simulink model "system_MW"  (R2023b)
settings: Solver=VariableStepAuto  StartTime=0.0  StopTime=0.3  MaxStep=1e-3  RelTol=1e-3  AbsTol=1e-3  EnableMultiTasking=on
values from neighbouring files (symbols this model uses):
  Ts = ts(k)    [example_MW.m]
  Un = 400    [example_MW.m]
undefined symbols (not defined in the file or in its folder): P
libraries: fl_lib x41, nesl_utility x27, ee_lib x19, eeGeneralControl x8
(part 1 of 2)
settings Model: Creator=neugebch  LastModifiedBy=neugebch
settings SolverCC: AutoScaleAbsTol=off  AlgebraicLoopSolver=TrustRegion  MaxZcPerStep=1
settings DataIOCC: LimitDataPoints=on  MaxDataPoints=10000
settings OptimizationCC: ReuseModelBlockBuffer=off  LifeSpan=inf
settings DebuggingCC: UnconnectedInputMsg=warning  UnconnectedOutputMsg=warning  UnconnectedLineMsg=warning  AllowSymbolicDim=off  SFUnexpectedBacktrackingDiag=warning  SFNoUnconditionalDefaultTransitionDiag=warning  SFExecutionAtInitializationDiag=none  ArithmeticOperatorsInVariantConditions=warning
settings ModelReferenceCC: EnableRefExpFcnMdlSchedulingChecks=on
settings SFSimCC: SimUseLocalCustomCode=off  CustomCodeUndefinedFunction=UseInterfaceOnly
settings RTWCC: RTWUseLocalCustomCode=off  DLArmComputeVersion=19.05
settings CodeAppCC: StateflowObjectComments=on
settings GRTTargetCC: TargetLangStandard=C89/C90 (ANSI)
settings ConfigComp: CovMetricSettings=dw  CovSaveCumulativeToWorkspaceVar=on  CovSaveSingleToWorkspaceVar=on  CovExternalEMLEnable=off  CovSFcnEnable=off
settings SimscapeCC: SimscapeLogType=all  SimscapeLogSimulationStatistics=on  SimscapeLogDataHistory=10000

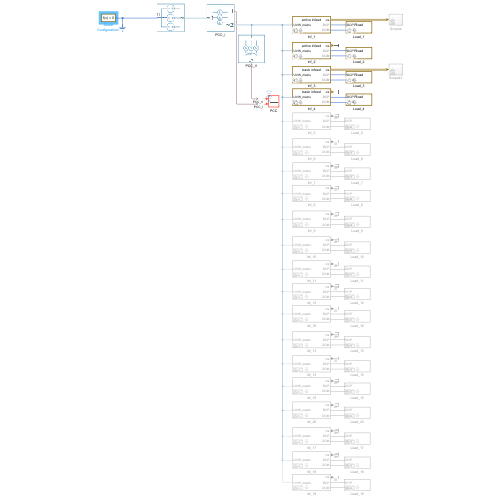
[thumbnail: Simulink's stored preview of the top-level diagram]
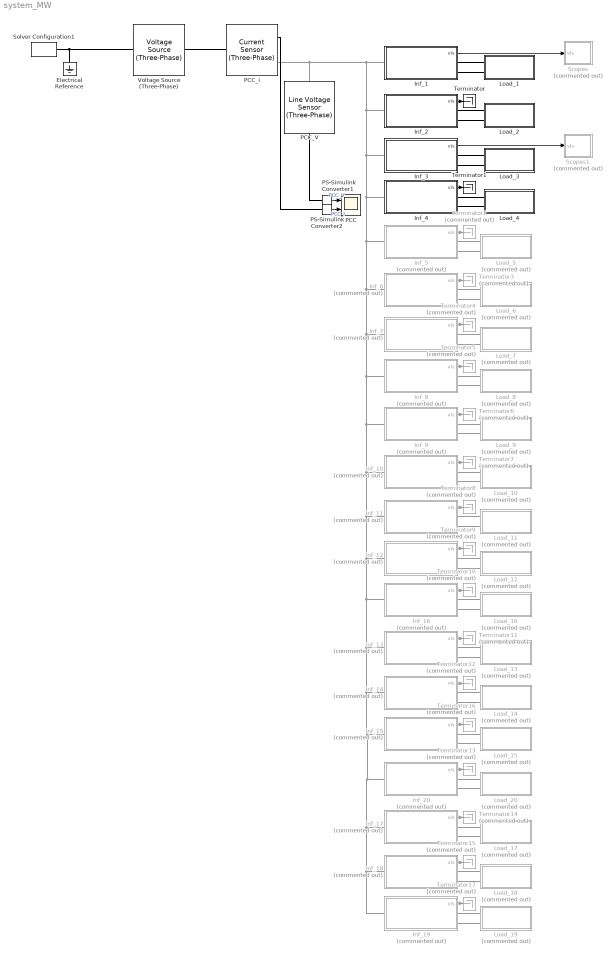
== system system_MW ==
  Electrical Reference : fl_lib/Electrical/Electrical Elements/Electrical Reference
  Inf_1 : Subsystem  Variant=on  mask{P=P(1), Ts=Ts}
  Inf_10 : Subsystem  Commented=on  Variant=on  mask{P=P(10), Ts=Ts}
  Inf_11 : Subsystem  Commented=on  Variant=on  mask{P=P(11), Ts=Ts}
  Inf_12 : Subsystem  Commented=on  Variant=on  mask{P=P(12), Ts=Ts}
  Inf_13 : Subsystem  Commented=on  Variant=on  mask{P=P(14), Ts=Ts}
  Inf_14 : Subsystem  Commented=on  Variant=on  mask{P=P(15), Ts=Ts}
  Inf_15 : Subsystem  Commented=on  Variant=on  mask{P=P(16), Ts=Ts}
  Inf_16 : Subsystem  Commented=on  Variant=on  mask{P=P(13), Ts=Ts}
  Inf_17 : Subsystem  Commented=on  Variant=on  mask{P=P(18), Ts=Ts}
  Inf_18 : Subsystem  Commented=on  Variant=on  mask{P=P(19), Ts=Ts}
  Inf_19 : Subsystem  Commented=on  Variant=on  mask{P=P(20), Ts=Ts}
  Inf_2 : Subsystem  Variant=on  mask{P=P(2), Ts=Ts}
  Inf_20 : Subsystem  Commented=on  Variant=on  mask{P=P(17), Ts=Ts}
  Inf_3 : Subsystem  Variant=on  mask{P=P(3), Ts=Ts}
  Inf_4 : Subsystem  Variant=on  mask{P=P(4), Ts=Ts}
  Inf_5 : Subsystem  Commented=on  Variant=on  mask{P=P(5), Ts=Ts}
  Inf_6 : Subsystem  Commented=on  Variant=on  mask{P=P(6), Ts=Ts}
  Inf_7 : Subsystem  Commented=on  Variant=on  mask{P=P(7), Ts=Ts}
  Inf_8 : Subsystem  Commented=on  Variant=on  mask{P=P(8), Ts=Ts}
  Inf_9 : Subsystem  Commented=on  Variant=on  mask{P=P(9), Ts=Ts}
  Load_1 : Subsystem  Variant=on  mask{P=P(1)}
  Load_10 : Subsystem  Commented=on  Variant=on  mask{P=P(10)}
  Load_11 : Subsystem  Commented=on  Variant=on  mask{P=P(11)}
  Load_12 : Subsystem  Commented=on  Variant=on  mask{P=P(12)}
  Load_13 : Subsystem  Commented=on  Variant=on  mask{P=P(14)}
  Load_14 : Subsystem  Commented=on  Variant=on  mask{P=P(15)}
  Load_15 : Subsystem  Commented=on  Variant=on  mask{P=P(16)}
  Load_16 : Subsystem  Commented=on  Variant=on  mask{P=P(13)}
  Load_17 : Subsystem  Commented=on  Variant=on  mask{P=P(18)}
  Load_18 : Subsystem  Commented=on  Variant=on  mask{P=P(19)}
  Load_19 : Subsystem  Commented=on  Variant=on  mask{P=P(20)}
  Load_2 : Subsystem  Variant=on  mask{P=P(2)}
  Load_20 : Subsystem  Commented=on  Variant=on  mask{P=P(17)}
  Load_3 : Subsystem  Variant=on  mask{P=P(3)}
  Load_4 : Subsystem  Variant=on  mask{P=P(4)}
  Load_5 : Subsystem  Commented=on  Variant=on  mask{P=P(5)}
  Load_6 : Subsystem  Commented=on  Variant=on  mask{P=P(6)}
  Load_7 : Subsystem  Commented=on  Variant=on  mask{P=P(7)}
  Load_8 : Subsystem  Commented=on  Variant=on  mask{P=P(8)}
  Load_9 : Subsystem  Commented=on  Variant=on  mask{P=P(9)}
  PCC : Scope  NumInputPorts=2
  PCC_V : ee_lib/Sensors & Transducers/Line Voltage Sensor (Three-Phase)
      settings: LogSimulationData=on
  PCC_i : ee_lib/Sensors & Transducers/Current Sensor (Three-Phase)
      settings: LogSimulationData=on
  PS-Simulink Converter1 : nesl_utility/PS-Simulink Converter  PhysicalDomain=network_engine_domain  SubClassName=ps_output  LeftPortType=input  RightPortType=output  PseudoPeriodic=off  Frequencies=[]  VectorFormat=inherit  Unit=inherit  AffineConversion=off
  PS-Simulink Converter2 : nesl_utility/PS-Simulink Converter  PhysicalDomain=network_engine_domain  SubClassName=ps_output  LeftPortType=input  RightPortType=output  PseudoPeriodic=off  Frequencies=[]  VectorFormat=inherit  Unit=inherit  AffineConversion=off
  Scopes : Subsystem  Commented=on
  Scopes1 : Subsystem  Commented=on
  Solver Configuration1 : nesl_utility/Solver Configuration  PhysicalDomain=network_engine_domain  SubClassName=solver  LeftPortType=input  RightPortType=generic  Tones=[]  Harmonics=[]  SimulateNoise=off  Profile=off  UseLocalSampling=off  EnableSwitchedLinearOptims=on  FrequencyDomain=off  UseCCode=off  RelTol=0.001  AbsTol=1e-06  MinStep=1e-09  ToWorkspace=off  RevertToSquareIcSolve=off  NumHomotopyIterations=100  PhasorMode=off  PhasorModeNumHarmonics=1  ConsistencySolver=NEWTON_FTOL  IndexReductionMethod=DerivativeReplacement  DoDC=off  ResidualTolerance=1e-09  ConsistencyTolSource=GLOBAL  ConsistencyAbsTol=0.001  ConsistencyRelTol=0.001  ConsistencyTolFactor=0.001  UseLocalSolver=on  LocalSolverChoice=NE_TRAPEZOIDAL_ADVANCER  ResolveIndetEquations=on  FunctionEvalNumThread=1  LocalSolverSampleTime=Ts  DoFixedCost=on  MaxNonlinIter=5  MaxModeIter=2  ComputeImpulses=off  ImpulseIterations=1  LinearAlgebra=auto  LinearAlgebraNumThread=0  EquationFormulation=NE_TIME_EF  DelaysMemoryBudget=1024  AutomaticFiltering=on  FilteringTimeConstant=0.001  PartitionStorageMethod=AS_NEEDED  PartitionMemoryBudget=1024  PartitionMethod=ROBUST  MultibodyUseLocalSolver=off  MultibodyLocalSolverChoice=ODE1  MultibodyLocalSolverSampleTime=0.001
  Terminator : Terminator
  Terminator1 : Terminator
  Terminator{2..17} (16 alike) : Terminator  Commented=on
  Voltage Source (Three-Phase) : ee_lib/Sources/Voltage Source (Three-Phase)  vline_rms=sqrt(3/2) * Un V  shift=0 deg  freq=fn Hz  impedance_option=1  SShortCircuit=Skv A*V  XR=X_R  R=0.01 Ohm  L=3.97e-4 H  harmonic_option=0  harmonic_orders=[5, 7, 11, 13]  harmonic_ratios=[.1, .1, .1, .1]  G_parasitic=0 1/Ohm  I_specify=off  I_priority=None  I=[0, 0, 0] A  I_nominal_specify=off  I_nominal_unit=A  I_nominal_value=1
  wires:
  Inf_1/1(vis) -> Scopes/1(vis)
  Inf_3/1(vis) -> Scopes1/1(vis)
  PS-Simulink Converter1/1 -> PCC/1  "PCC_V"
  PS-Simulink Converter2/1 -> PCC/2  "PCC_I"
  Inf_2/1(vis) -> Terminator/1
  Inf_4/1(vis) -> Terminator1/1
  Inf_5/1(vis) -> Terminator2/1
  Inf_6/1(vis) -> Terminator3/1
  Inf_7/1(vis) -> Terminator4/1
  Inf_8/1(vis) -> Terminator5/1
  Inf_9/1(vis) -> Terminator6/1
  Inf_10/1(vis) -> Terminator7/1
  Inf_11/1(vis) -> Terminator8/1
  Inf_12/1(vis) -> Terminator9/1
  Inf_16/1(vis) -> Terminator10/1
  Inf_13/1(vis) -> Terminator11/1
  Inf_14/1(vis) -> Terminator12/1
  Inf_15/1(vis) -> Terminator16/1
  Inf_20/1(vis) -> Terminator13/1
  Inf_17/1(vis) -> Terminator14/1
  Inf_18/1(vis) -> Terminator15/1
  Inf_19/1(vis) -> Terminator17/1
  connections:
  Solver Configuration1/RConn1 -- Voltage Source (Three-Phase)/LConn1 -- Electrical Reference/LConn1
  Inf_18/LConn1 -- Inf_20/LConn1 -- Inf_14/LConn1 -- Inf_13/LConn1 -- Inf_10/LConn1 -- Inf_7/LConn1 -- Inf_2/LConn1 -- PCC_V/LConn1 -- PCC_i/RConn2 -- Inf_1/LConn1 -- Inf_3/LConn1 -- Inf_4/LConn1 -- Inf_5/LConn1 -- Inf_6/LConn1 -- Inf_8/LConn1 -- Inf_9/LConn1 -- Inf_11/LConn1 -- Inf_12/LConn1 -- Inf_16/LConn1 -- Inf_15/LConn1 -- Inf_17/LConn1 -- Inf_19/LConn1
  PS-Simulink Converter1/LConn1 -- PCC_V/RConn1
  Load_1/LConn1 -- Inf_1/RConn1
  Load_1/LConn2 -- Inf_1/RConn2
  Load_2/LConn1 -- Inf_2/RConn1
  Load_2/LConn2 -- Inf_2/RConn2
  Load_3/LConn1 -- Inf_3/RConn1
  Load_3/LConn2 -- Inf_3/RConn2
  Voltage Source (Three-Phase)/RConn1 -- PCC_i/LConn1
  PS-Simulink Converter2/LConn1 -- PCC_i/RConn1
  Load_4/LConn2 -- Inf_4/RConn2
  Load_4/LConn1 -- Inf_4/RConn1
  Load_8/LConn1 -- Inf_8/RConn1
  Load_6/LConn2 -- Inf_6/RConn2
  Inf_5/RConn2 -- Load_5/LConn2
  Load_6/LConn1 -- Inf_6/RConn1
  Load_7/LConn2 -- Inf_7/RConn2
  Load_8/LConn2 -- Inf_8/RConn2
  Inf_5/RConn1 -- Load_5/LConn1
  Load_7/LConn1 -- Inf_7/RConn1
  Load_11/LConn1 -- Inf_11/RConn1
  Inf_9/RConn1 -- Load_9/LConn1
  Load_10/LConn1 -- Inf_10/RConn1
  Load_12/LConn2 -- Inf_12/RConn2
  Load_11/LConn2 -- Inf_11/RConn2
  Inf_9/RConn2 -- Load_9/LConn2
  Load_12/LConn1 -- Inf_12/RConn1
  Load_10/LConn2 -- Inf_10/RConn2
  Load_13/LConn2 -- Inf_13/RConn2
  Load_15/LConn1 -- Inf_15/RConn1
  Load_14/LConn2 -- Inf_14/RConn2
  Inf_16/RConn2 -- Load_16/LConn2
  Load_15/LConn2 -- Inf_15/RConn2
  Load_13/LConn1 -- Inf_13/RConn1
  Load_14/LConn1 -- Inf_14/RConn1
  Inf_16/RConn1 -- Load_16/LConn1
  Inf_20/RConn1 -- Load_20/LConn1
  Load_19/LConn2 -- Inf_19/RConn2
  Inf_20/RConn2 -- Load_20/LConn2
  Load_17/LConn1 -- Inf_17/RConn1
  Load_18/LConn2 -- Inf_18/RConn2
  Load_17/LConn2 -- Inf_17/RConn2
  Load_19/LConn1 -- Inf_19/RConn1
  Load_18/LConn1 -- Inf_18/RConn1

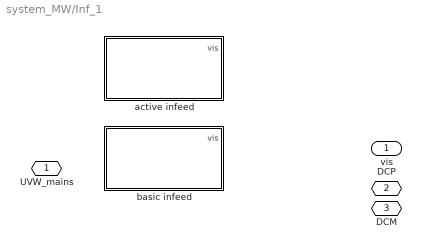
== system system_MW/Inf_1 ==
  active infeed : Subsystem  Variant=on  VariantControlMode=label  VariantControl=true  LabelModeActiveChoice=Choice
  basic infeed : Subsystem  Variant=on  VariantControlMode=label  VariantControl=false  LabelModeActiveChoice=Choice_1
  UVW_mains : PMIOPort  Side=Left
  DCP : PMIOPort  Port=2  Side=Right
  DCM : PMIOPort  Port=3  Side=Right
  vis : Outport

== system system_MW/Inf_10 ==
  active infeed : Subsystem  VariantControl=true  ReferencedSubsystem=active_infeed  P=P  Ts=Ts
  basic infeed : Subsystem  VariantControl=false  ReferencedSubsystem=basic_infeed  P=P  Ts=Ts
  UVW_mains : PMIOPort  Side=Left
  DCP : PMIOPort  Port=2  Side=Right
  DCM : PMIOPort  Port=3  Side=Right
  vis : Outport

== system system_MW/Inf_11 ==
  active infeed : Subsystem  VariantControl=false  ReferencedSubsystem=active_infeed  P=P  Ts=Ts
  basic infeed : Subsystem  VariantControl=true  ReferencedSubsystem=basic_infeed  P=P  Ts=Ts
  UVW_mains : PMIOPort  Side=Left
  DCP : PMIOPort  Port=2  Side=Right
  DCM : PMIOPort  Port=3  Side=Right
  vis : Outport

== system system_MW/Inf_12 ==
  active infeed : Subsystem  VariantControl=false  ReferencedSubsystem=active_infeed  P=P  Ts=Ts
  basic infeed : Subsystem  VariantControl=true  ReferencedSubsystem=basic_infeed  P=P  Ts=Ts
  UVW_mains : PMIOPort  Side=Left
  DCP : PMIOPort  Port=2  Side=Right
  DCM : PMIOPort  Port=3  Side=Right
  vis : Outport

== system system_MW/Inf_13 ==
  active infeed : Subsystem  VariantControl=true  ReferencedSubsystem=active_infeed  P=P  Ts=Ts
  basic infeed : Subsystem  VariantControl=false  ReferencedSubsystem=basic_infeed  P=P  Ts=Ts
  UVW_mains : PMIOPort  Side=Left
  DCP : PMIOPort  Port=2  Side=Right
  DCM : PMIOPort  Port=3  Side=Right
  vis : Outport

== system system_MW/Inf_14 ==
  active infeed : Subsystem  VariantControl=false  ReferencedSubsystem=active_infeed  P=P  Ts=Ts
  basic infeed : Subsystem  VariantControl=true  ReferencedSubsystem=basic_infeed  P=P  Ts=Ts
  UVW_mains : PMIOPort  Side=Left
  DCP : PMIOPort  Port=2  Side=Right
  DCM : PMIOPort  Port=3  Side=Right
  vis : Outport

== system system_MW/Inf_15 ==
  active infeed : Subsystem  VariantControl=false  ReferencedSubsystem=active_infeed  P=P  Ts=Ts
  basic infeed : Subsystem  VariantControl=true  ReferencedSubsystem=basic_infeed  P=P  Ts=Ts
  UVW_mains : PMIOPort  Side=Left
  DCP : PMIOPort  Port=2  Side=Right
  DCM : PMIOPort  Port=3  Side=Right
  vis : Outport

== system system_MW/Inf_16 ==
  active infeed : Subsystem  Variant=on  VariantControlMode=label  VariantControl=true  LabelModeActiveChoice=Choice
  basic infeed : Subsystem  Variant=on  VariantControlMode=label  VariantControl=false  LabelModeActiveChoice=Choice_1
  UVW_mains : PMIOPort  Side=Left
  DCP : PMIOPort  Port=2  Side=Right
  DCM : PMIOPort  Port=3  Side=Right
  vis : Outport

== system system_MW/Inf_17 ==
  active infeed : Subsystem  VariantControl=true  ReferencedSubsystem=active_infeed  P=P  Ts=Ts
  basic infeed : Subsystem  VariantControl=false  ReferencedSubsystem=basic_infeed  P=P  Ts=Ts
  UVW_mains : PMIOPort  Side=Left
  DCP : PMIOPort  Port=2  Side=Right
  DCM : PMIOPort  Port=3  Side=Right
  vis : Outport

== system system_MW/Inf_18 ==
  active infeed : Subsystem  VariantControl=false  ReferencedSubsystem=active_infeed  P=P  Ts=Ts
  basic infeed : Subsystem  VariantControl=true  ReferencedSubsystem=basic_infeed  P=P  Ts=Ts
  UVW_mains : PMIOPort  Side=Left
  DCP : PMIOPort  Port=2  Side=Right
  DCM : PMIOPort  Port=3  Side=Right
  vis : Outport

== system system_MW/Inf_19 ==
  active infeed : Subsystem  VariantControl=false  ReferencedSubsystem=active_infeed  P=P  Ts=Ts
  basic infeed : Subsystem  VariantControl=true  ReferencedSubsystem=basic_infeed  P=P  Ts=Ts
  UVW_mains : PMIOPort  Side=Left
  DCP : PMIOPort  Port=2  Side=Right
  DCM : PMIOPort  Port=3  Side=Right
  vis : Outport

== system system_MW/Inf_2 ==
  active infeed : Subsystem  VariantControl=true  ReferencedSubsystem=active_infeed  P=P  Ts=Ts
  basic infeed : Subsystem  VariantControl=false  ReferencedSubsystem=basic_infeed  P=P  Ts=Ts
  UVW_mains : PMIOPort  Side=Left
  DCP : PMIOPort  Port=2  Side=Right
  DCM : PMIOPort  Port=3  Side=Right
  vis : Outport

== system system_MW/Inf_20 ==
  active infeed : Subsystem  Variant=on  VariantControlMode=label  VariantControl=true  LabelModeActiveChoice=Choice
  basic infeed : Subsystem  Variant=on  VariantControlMode=label  VariantControl=false  LabelModeActiveChoice=Choice_1
  UVW_mains : PMIOPort  Side=Left
  DCP : PMIOPort  Port=2  Side=Right
  DCM : PMIOPort  Port=3  Side=Right
  vis : Outport

== system system_MW/Inf_3 ==
  active infeed : Subsystem  VariantControl=false  ReferencedSubsystem=active_infeed  P=P  Ts=Ts
  basic infeed : Subsystem  VariantControl=true  ReferencedSubsystem=basic_infeed  P=P  Ts=Ts
  UVW_mains : PMIOPort  Side=Left
  DCP : PMIOPort  Port=2  Side=Right
  DCM : PMIOPort  Port=3  Side=Right
  vis : Outport

== system system_MW/Inf_4 ==
  active infeed : Subsystem  VariantControl=false  ReferencedSubsystem=active_infeed  P=P  Ts=Ts
  basic infeed : Subsystem  VariantControl=true  ReferencedSubsystem=basic_infeed  P=P  Ts=Ts
  UVW_mains : PMIOPort  Side=Left
  DCP : PMIOPort  Port=2  Side=Right
  DCM : PMIOPort  Port=3  Side=Right
  vis : Outport

== system system_MW/Inf_5 ==
  active infeed : Subsystem  Variant=on  VariantControlMode=label  VariantControl=true  LabelModeActiveChoice=Choice
  basic infeed : Subsystem  Variant=on  VariantControlMode=label  VariantControl=false  LabelModeActiveChoice=Choice_1
  UVW_mains : PMIOPort  Side=Left
  DCP : PMIOPort  Port=2  Side=Right
  DCM : PMIOPort  Port=3  Side=Right
  vis : Outport

== system system_MW/Inf_6 ==
  active infeed : Subsystem  VariantControl=true  ReferencedSubsystem=active_infeed  P=P  Ts=Ts
  basic infeed : Subsystem  VariantControl=false  ReferencedSubsystem=basic_infeed  P=P  Ts=Ts
  UVW_mains : PMIOPort  Side=Left
  DCP : PMIOPort  Port=2  Side=Right
  DCM : PMIOPort  Port=3  Side=Right
  vis : Outport

== system system_MW/Inf_7 ==
  active infeed : Subsystem  VariantControl=false  ReferencedSubsystem=active_infeed  P=P  Ts=Ts
  basic infeed : Subsystem  VariantControl=true  ReferencedSubsystem=basic_infeed  P=P  Ts=Ts
  UVW_mains : PMIOPort  Side=Left
  DCP : PMIOPort  Port=2  Side=Right
  DCM : PMIOPort  Port=3  Side=Right
  vis : Outport

== system system_MW/Inf_8 ==
  active infeed : Subsystem  VariantControl=false  ReferencedSubsystem=active_infeed  P=P  Ts=Ts
  basic infeed : Subsystem  VariantControl=true  ReferencedSubsystem=basic_infeed  P=P  Ts=Ts
  UVW_mains : PMIOPort  Side=Left
  DCP : PMIOPort  Port=2  Side=Right
  DCM : PMIOPort  Port=3  Side=Right
  vis : Outport

== system system_MW/Inf_9 ==
  active infeed : Subsystem  Variant=on  VariantControlMode=label  VariantControl=true  LabelModeActiveChoice=Choice
  basic infeed : Subsystem  Variant=on  VariantControlMode=label  VariantControl=false  LabelModeActiveChoice=Choice_1
  UVW_mains : PMIOPort  Side=Left
  DCP : PMIOPort  Port=2  Side=Right
  DCM : PMIOPort  Port=3  Side=Right
  vis : Outport

== system system_MW/Load_1 ==
  Rload : Subsystem  VariantControl=true  ReferencedSubsystem=Rload
  Vdc : Subsystem  VariantControl=false  ReferencedSubsystem=Vdc
  DCP : PMIOPort  Side=Left
  DCM : PMIOPort  Port=2  Side=Left

== system system_MW/Load_10 ==
  Rload : Subsystem  VariantControl=true
  Vdc : Subsystem  VariantControl=false
  DCP : PMIOPort  Side=Left
  DCM : PMIOPort  Port=2  Side=Left

== system system_MW/Load_11 ==
  Rload : Subsystem  VariantControl=true
  Vdc : Subsystem  VariantControl=false
  DCP : PMIOPort  Side=Left
  DCM : PMIOPort  Port=2  Side=Left

== system system_MW/Load_12 ==
  Rload : Subsystem  VariantControl=true
  Vdc : Subsystem  VariantControl=false
  DCP : PMIOPort  Side=Left
  DCM : PMIOPort  Port=2  Side=Left

== system system_MW/Load_13 ==
  Rload : Subsystem  VariantControl=true
  Vdc : Subsystem  VariantControl=false
  DCP : PMIOPort  Side=Left
  DCM : PMIOPort  Port=2  Side=Left

== system system_MW/Load_14 ==
  Rload : Subsystem  VariantControl=true
  Vdc : Subsystem  VariantControl=false
  DCP : PMIOPort  Side=Left
  DCM : PMIOPort  Port=2  Side=Left

== system system_MW/Load_15 ==
  Rload : Subsystem  VariantControl=true
  Vdc : Subsystem  VariantControl=false
  DCP : PMIOPort  Side=Left
  DCM : PMIOPort  Port=2  Side=Left

== system system_MW/Load_16 ==
  Rload : Subsystem  VariantControl=true
  Vdc : Subsystem  VariantControl=false
  DCP : PMIOPort  Side=Left
  DCM : PMIOPort  Port=2  Side=Left

== system system_MW/Load_17 ==
  Rload : Subsystem  VariantControl=true
  Vdc : Subsystem  VariantControl=false
  DCP : PMIOPort  Side=Left
  DCM : PMIOPort  Port=2  Side=Left

== system system_MW/Load_18 ==
  Rload : Subsystem  VariantControl=true
  Vdc : Subsystem  VariantControl=false
  DCP : PMIOPort  Side=Left
  DCM : PMIOPort  Port=2  Side=Left

== system system_MW/Load_19 ==
  Rload : Subsystem  VariantControl=true
  Vdc : Subsystem  VariantControl=false
  DCP : PMIOPort  Side=Left
  DCM : PMIOPort  Port=2  Side=Left

== system system_MW/Load_2 ==
  Rload : Subsystem  VariantControl=true  ReferencedSubsystem=Rload
  Vdc : Subsystem  VariantControl=false  ReferencedSubsystem=Vdc
  DCP : PMIOPort  Side=Left
  DCM : PMIOPort  Port=2  Side=Left

== system system_MW/Load_20 ==
  Rload : Subsystem  VariantControl=true
  Vdc : Subsystem  VariantControl=false
  DCP : PMIOPort  Side=Left
  DCM : PMIOPort  Port=2  Side=Left

== system system_MW/Load_3 ==
  Rload : Subsystem  VariantControl=true  ReferencedSubsystem=Rload
  Vdc : Subsystem  VariantControl=false  ReferencedSubsystem=Vdc
  DCP : PMIOPort  Side=Left
  DCM : PMIOPort  Port=2  Side=Left

== system system_MW/Load_4 ==
  Rload : Subsystem  VariantControl=true  ReferencedSubsystem=Rload
  Vdc : Subsystem  VariantControl=false  ReferencedSubsystem=Vdc
  DCP : PMIOPort  Side=Left
  DCM : PMIOPort  Port=2  Side=Left

== system system_MW/Load_5 ==
  Rload : Subsystem  VariantControl=true
  Vdc : Subsystem  VariantControl=false
  DCP : PMIOPort  Side=Left
  DCM : PMIOPort  Port=2  Side=Left

== system system_MW/Load_6 ==
  Rload : Subsystem  VariantControl=true
  Vdc : Subsystem  VariantControl=false
  DCP : PMIOPort  Side=Left
  DCM : PMIOPort  Port=2  Side=Left

== system system_MW/Load_7 ==
  Rload : Subsystem  VariantControl=true
  Vdc : Subsystem  VariantControl=false
  DCP : PMIOPort  Side=Left
  DCM : PMIOPort  Port=2  Side=Left

== system system_MW/Load_8 ==
  Rload : Subsystem  VariantControl=true
  Vdc : Subsystem  VariantControl=false
  DCP : PMIOPort  Side=Left
  DCM : PMIOPort  Port=2  Side=Left

== system system_MW/Load_9 ==
  Rload : Subsystem  VariantControl=true
  Vdc : Subsystem  VariantControl=false
  DCP : PMIOPort  Side=Left
  DCM : PMIOPort  Port=2  Side=Left

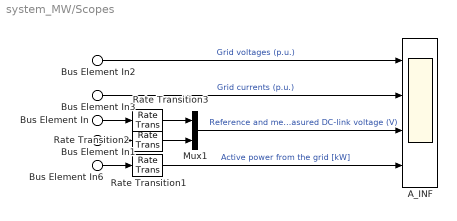
== system system_MW/Scopes ==
  Bus Element In : Inport  PortName=vis  Element=VdcRef
  Bus Element In1 : Inport  PortName=vis  Element=VdcF
  Bus Element In2 : Inport  PortName=vis  Element=VgABC
  Bus Element In3 : Inport  PortName=vis  Element=IgABC
  Bus Element In6 : Inport  PortName=vis  Element=Pt
  A_INF : Scope  NumInputPorts=4
  Mux1 : Mux  Inputs=2
  Rate Transition1 : RateTransition
  Rate Transition2 : RateTransition
  Rate Transition3 : RateTransition
  wires:
  Rate Transition2/1 -> Mux1/2
  Bus Element In/1 -> Rate Transition3/1
  Mux1/1 -> A_INF/3  "Reference and measured DC-link voltage (V)"
  Bus Element In2/1 -> A_INF/1  "Grid voltages (p.u.)"
  Bus Element In3/1 -> A_INF/2  "Grid currents (p.u.)"
  Rate Transition1/1 -> A_INF/4  "Active power from the grid [kW]"
  Bus Element In1/1 -> Rate Transition2/1
  Rate Transition3/1 -> Mux1/1
  Bus Element In6/1 -> Rate Transition1/1

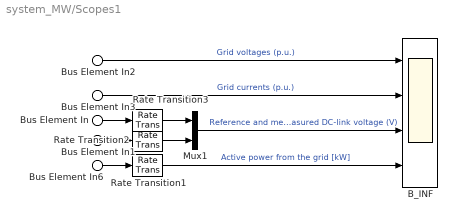
== system system_MW/Scopes1 ==
  Bus Element In : Inport  PortName=vis  Element=VdcRef
  Bus Element In1 : Inport  PortName=vis  Element=VdcF
  Bus Element In2 : Inport  PortName=vis  Element=VgABC
  Bus Element In3 : Inport  PortName=vis  Element=IgABC
  Bus Element In6 : Inport  PortName=vis  Element=Pt
  B_INF : Scope  NumInputPorts=4
  Mux1 : Mux  Inputs=2
  Rate Transition1 : RateTransition
  Rate Transition2 : RateTransition
  Rate Transition3 : RateTransition
  wires:
  Bus Element In6/1 -> Rate Transition1/1
  Rate Transition3/1 -> Mux1/1
  Bus Element In1/1 -> Rate Transition2/1
  Rate Transition1/1 -> B_INF/4  "Active power from the grid [kW]"
  Bus Element In3/1 -> B_INF/2  "Grid currents (p.u.)"
  Bus Element In2/1 -> B_INF/1  "Grid voltages (p.u.)"
  Mux1/1 -> B_INF/3  "Reference and measured DC-link voltage (V)"
  Bus Element In/1 -> Rate Transition3/1
  Rate Transition2/1 -> Mux1/2

== system system_MW/Inf_1/active infeed ==
  active infeed : Subsystem  VariantControl=Choice  ReferencedSubsystem=active_infeed  P=P  Ts=Ts
  UVW_mains : PMIOPort  Side=Left
  DCP : PMIOPort  Port=2  Side=Right
  DCM : PMIOPort  Port=3  Side=Right
  vis : Outport

== system system_MW/Inf_1/basic infeed ==
  basic infeed : Subsystem  VariantControl=Choice_1  ReferencedSubsystem=basic_infeed  P=P  Ts=Ts
  UVW_mains : PMIOPort  Side=Left
  DCP : PMIOPort  Port=2  Side=Right
  DCM : PMIOPort  Port=3  Side=Right
  vis : Outport

== system system_MW/Inf_16/active infeed ==
  active infeed : Subsystem  VariantControl=Choice  ReferencedSubsystem=active_infeed  P=P  Ts=Ts
  UVW_mains : PMIOPort  Side=Left
  DCP : PMIOPort  Port=2  Side=Right
  DCM : PMIOPort  Port=3  Side=Right
  vis : Outport

== system system_MW/Inf_16/basic infeed ==
  basic infeed : Subsystem  VariantControl=Choice_1  ReferencedSubsystem=basic_infeed  P=P  Ts=Ts
  UVW_mains : PMIOPort  Side=Left
  DCP : PMIOPort  Port=2  Side=Right
  DCM : PMIOPort  Port=3  Side=Right
  vis : Outport

== system system_MW/Inf_20/active infeed ==
  active infeed : Subsystem  VariantControl=Choice  ReferencedSubsystem=active_infeed  P=P  Ts=Ts
  UVW_mains : PMIOPort  Side=Left
  DCP : PMIOPort  Port=2  Side=Right
  DCM : PMIOPort  Port=3  Side=Right
  vis : Outport

== system system_MW/Inf_20/basic infeed ==
  basic infeed : Subsystem  VariantControl=Choice_1  ReferencedSubsystem=basic_infeed  P=P  Ts=Ts
  UVW_mains : PMIOPort  Side=Left
  DCP : PMIOPort  Port=2  Side=Right
  DCM : PMIOPort  Port=3  Side=Right
  vis : Outport

== system system_MW/Inf_5/active infeed ==
  active infeed : Subsystem  VariantControl=Choice  ReferencedSubsystem=active_infeed  P=P  Ts=Ts
  UVW_mains : PMIOPort  Side=Left
  DCP : PMIOPort  Port=2  Side=Right
  DCM : PMIOPort  Port=3  Side=Right
  vis : Outport

== system system_MW/Inf_5/basic infeed ==
  basic infeed : Subsystem  VariantControl=Choice_1  ReferencedSubsystem=basic_infeed  P=P  Ts=Ts
  UVW_mains : PMIOPort  Side=Left
  DCP : PMIOPort  Port=2  Side=Right
  DCM : PMIOPort  Port=3  Side=Right
  vis : Outport

== system system_MW/Inf_9/active infeed ==
  active infeed : Subsystem  VariantControl=Choice  ReferencedSubsystem=active_infeed  P=P  Ts=Ts
  UVW_mains : PMIOPort  Side=Left
  DCP : PMIOPort  Port=2  Side=Right
  DCM : PMIOPort  Port=3  Side=Right
  vis : Outport

== system system_MW/Inf_9/basic infeed ==
  basic infeed : Subsystem  VariantControl=Choice_1  ReferencedSubsystem=basic_infeed  P=P  Ts=Ts
  UVW_mains : PMIOPort  Side=Left
  DCP : PMIOPort  Port=2  Side=Right
  DCM : PMIOPort  Port=3  Side=Right
  vis : Outport

== system system_MW/Load_10/Rload ==
  Resistor1 : fl_lib/Electrical/Electrical Elements/Resistor  R=P.Un/P.In/P.p Ohm  i_specify=off  i_priority=None  i=0 A  i_nominal_specify=off  i_nominal_unit=A  i_nominal_value=1  v_specify=off  v_priority=None  v=0 V  v_nominal_specify=off  v_nominal_unit=V  v_nominal_value=1
  DCP : PMIOPort  Side=Left
  DCM : PMIOPort  Port=2  Side=Left
  connections:
  DCM/RConn1 -- Resistor1/RConn1
  DCP/RConn1 -- Resistor1/LConn1

== system system_MW/Load_10/Vdc ==
  Voltage Source : ee_lib/Sources/Voltage Source  dc_voltage=P.Udc V  ac_voltage=0 V  ac_shift=0 rad  ac_frequency=fn Hz  noise_mode=ee.enum.sources.noise.Disabled  PSD=0 V^2/Hz  sample_time=1e-3 s  repeatability=ee.enum.sources.repeatability.NotRepeatable  user_seed=0  auto_seed=3346497771  i_specify=off  i_priority=None  i=0 A  i_nominal_specify=off  i_nominal_unit=A  i_nominal_value=1  v_specify=off  v_priority=None  v=0 V  v_nominal_specify=off  v_nominal_unit=V  v_nominal_value=1
  DCP : PMIOPort  Side=Left
  DCM : PMIOPort  Port=2  Side=Left
  connections:
  DCM/RConn1 -- Voltage Source/RConn1
  DCP/RConn1 -- Voltage Source/LConn1

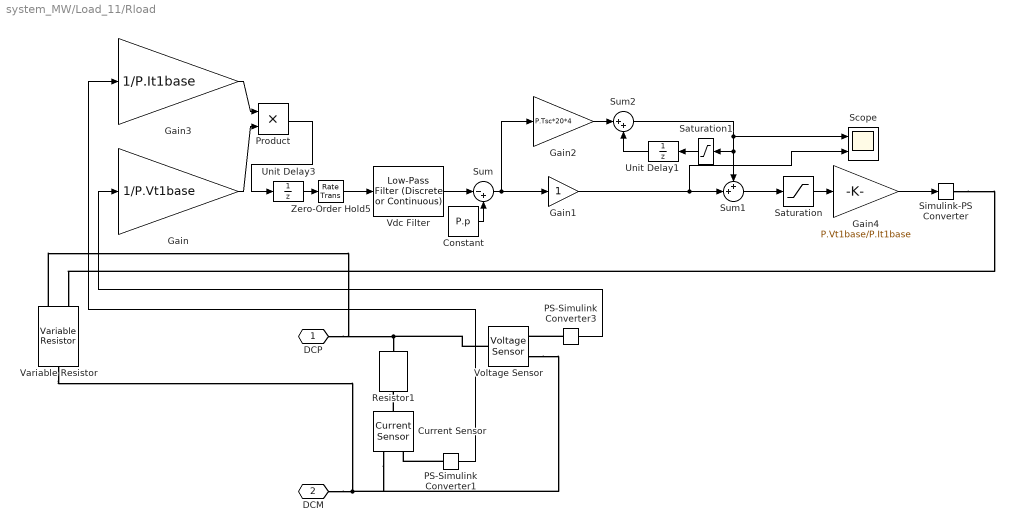
== system system_MW/Load_11/Rload ==
  Constant : Constant  Value=P.p
  Current Sensor : fl_lib/Electrical/Electrical Sensors/Current Sensor
  Gain : Gain  Gain=1/P.Vt1base
  Gain1 : Gain
  Gain2 : Gain  Gain=P.Tsc*20*4
  Gain3 : Gain  Gain=1/P.It1base
  Gain4 : Gain  Gain=P.Vt1base/P.It1base
  PS-Simulink Converter1 : nesl_utility/PS-Simulink Converter  PhysicalDomain=network_engine_domain  SubClassName=ps_output  LeftPortType=input  RightPortType=output  PseudoPeriodic=off  Frequencies=[]  VectorFormat=1-D array  Unit=1  AffineConversion=off
  PS-Simulink Converter3 : nesl_utility/PS-Simulink Converter  PhysicalDomain=network_engine_domain  SubClassName=ps_output  LeftPortType=input  RightPortType=output  PseudoPeriodic=off  Frequencies=[]  VectorFormat=1-D array  Unit=1  AffineConversion=off
  Product : Product
  Resistor1 : fl_lib/Electrical/Electrical Elements/Resistor  R=P.Un/P.In/P.p Ohm  i_specify=off  i_priority=None  i=0 A  i_nominal_specify=off  i_nominal_unit=A  i_nominal_value=1  v_specify=off  v_priority=None  v=0 V  v_nominal_specify=off  v_nominal_unit=V  v_nominal_value=1
  Saturation : Saturate  UpperLimit=10  LowerLimit=-10
  Saturation1 : Saturate  UpperLimit=10  LowerLimit=-10
  Scope : Scope  NumInputPorts=2
  Simulink-PS Converter : nesl_utility/Simulink-PS Converter  PhysicalDomain=network_engine_domain  SubClassName=ps_input  LeftPortType=input  RightPortType=output  PseudoPeriodic=off  Frequencies=[]  NoiseDistribution=none  NoiseParameters=[]  Unit=1  AffineConversion=off  FilteringAndDerivatives=provide  SimscapeFilterOrder=1  InputFilterTimeConstant=0.001  UdotUserProvided=0
  Sum : Sum  Inputs=|-+
  Sum1 : Sum  Inputs=++|
  Sum2 : Sum  Inputs=|++
  Unit Delay1 : UnitDelay  SampleTime=P.Tsc  HasFrameUpgradeWarning=on
  Unit Delay3 : UnitDelay  SampleTime=Ts  HasFrameUpgradeWarning=on
  Variable Resistor : fl_lib/Electrical/Electrical Elements/Variable Resistor  Rmin=0 Ohm  thermalEnable=false  thermal_mass=1 J/K  i_specify=off  i_priority=None  i=0 A  i_nominal_specify=off  i_nominal_unit=A  i_nominal_value=1  v_specify=off  v_priority=None  v=0 V  v_nominal_specify=off  v_nominal_unit=V  v_nominal_value=1  T_specify=off  T_priority=None  T=300 K  T_nominal_specify=off  T_nominal_unit=K  T_nominal_value=1
  Vdc Filter : eeGeneralControl/Low-Pass Filter (Discrete or Continuous)  K=1  T=1e-2  B=inf  A=-inf  init_option=Inherited from block input  x0=0  Ts=P.Tsc
  Voltage Sensor : fl_lib/Electrical/Electrical Sensors/Voltage Sensor
  Zero-Order Hold5 : RateTransition  OutPortSampleTime=P.Tsc
  DCP : PMIOPort  Side=Left
  DCM : PMIOPort  Port=2  Side=Left
  wires:
  Zero-Order Hold5/1 -> Vdc Filter/1
  PS-Simulink Converter3/1 -> Gain/1
  Unit Delay3/1 -> Zero-Order Hold5/1
  Vdc Filter/1 -> Sum/1
  Gain/1 -> Product/2
  Constant/1 -> Sum/2
  Sum1/1 -> Saturation/1
  Sum/1 -> Gain2/1, Gain1/1
  Sum2/1 -> Saturation1/1, Sum1/1, Scope/1
  Gain1/1 -> Scope/2, Sum1/2
  Gain2/1 -> Sum2/1
  Unit Delay1/1 -> Sum2/2
  PS-Simulink Converter1/1 -> Gain3/1
  Gain3/1 -> Product/1
  Product/1 -> Unit Delay3/1
  Saturation/1 -> Gain4/1
  Saturation1/1 -> Unit Delay1/1
  Gain4/1 -> Simulink-PS Converter/1
  connections:
  Voltage Sensor/LConn1 -- Resistor1/LConn1 -- DCP/RConn1 -- Variable Resistor/LConn2
  Variable Resistor/RConn1 -- DCM/RConn1 -- Voltage Sensor/RConn2 -- Current Sensor/RConn2
  PS-Simulink Converter3/LConn1 -- Voltage Sensor/RConn1
  Simulink-PS Converter/RConn1 -- Variable Resistor/LConn1
  Current Sensor/LConn1 -- Resistor1/RConn1
  PS-Simulink Converter1/LConn1 -- Current Sensor/RConn1

== system system_MW/Load_11/Vdc ==
  Voltage Source : ee_lib/Sources/Voltage Source  dc_voltage=P.Udc V  ac_voltage=0 V  ac_shift=0 rad  ac_frequency=fn Hz  noise_mode=ee.enum.sources.noise.Disabled  PSD=0 V^2/Hz  sample_time=1e-3 s  repeatability=ee.enum.sources.repeatability.NotRepeatable  user_seed=0  auto_seed=4011545342  i_specify=off  i_priority=None  i=0 A  i_nominal_specify=off  i_nominal_unit=A  i_nominal_value=1  v_specify=off  v_priority=None  v=0 V  v_nominal_specify=off  v_nominal_unit=V  v_nominal_value=1
  DCP : PMIOPort  Side=Left
  DCM : PMIOPort  Port=2  Side=Left
  connections:
  DCP/RConn1 -- Voltage Source/LConn1
  DCM/RConn1 -- Voltage Source/RConn1

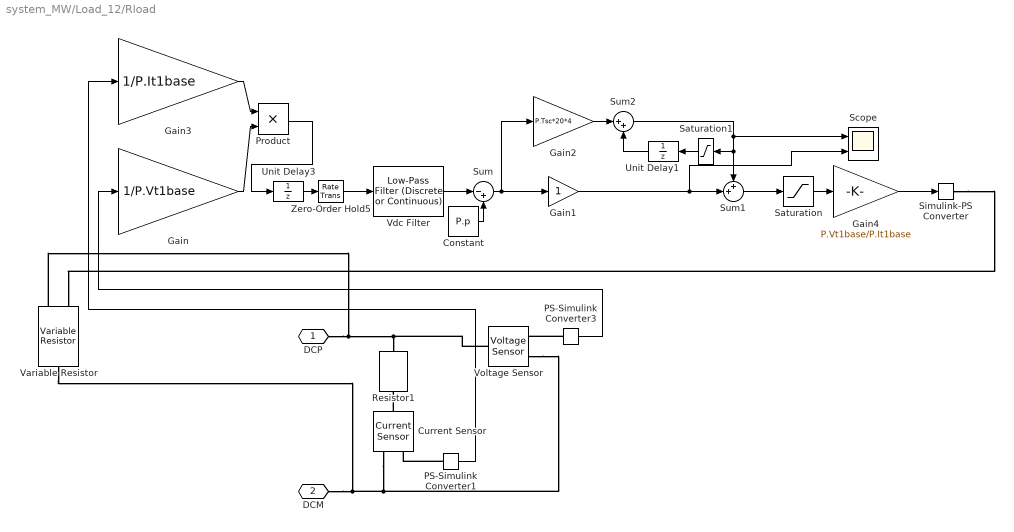
== system system_MW/Load_12/Rload ==
  Constant : Constant  Value=P.p
  Current Sensor : fl_lib/Electrical/Electrical Sensors/Current Sensor
  Gain : Gain  Gain=1/P.Vt1base
  Gain1 : Gain
  Gain2 : Gain  Gain=P.Tsc*20*4
  Gain3 : Gain  Gain=1/P.It1base
  Gain4 : Gain  Gain=P.Vt1base/P.It1base
  PS-Simulink Converter1 : nesl_utility/PS-Simulink Converter  PhysicalDomain=network_engine_domain  SubClassName=ps_output  LeftPortType=input  RightPortType=output  PseudoPeriodic=off  Frequencies=[]  VectorFormat=1-D array  Unit=1  AffineConversion=off
  PS-Simulink Converter3 : nesl_utility/PS-Simulink Converter  PhysicalDomain=network_engine_domain  SubClassName=ps_output  LeftPortType=input  RightPortType=output  PseudoPeriodic=off  Frequencies=[]  VectorFormat=1-D array  Unit=1  AffineConversion=off
  Product : Product
  Resistor1 : fl_lib/Electrical/Electrical Elements/Resistor  R=P.Un/P.In/P.p Ohm  i_specify=off  i_priority=None  i=0 A  i_nominal_specify=off  i_nominal_unit=A  i_nominal_value=1  v_specify=off  v_priority=None  v=0 V  v_nominal_specify=off  v_nominal_unit=V  v_nominal_value=1
  Saturation : Saturate  UpperLimit=10  LowerLimit=-10
  Saturation1 : Saturate  UpperLimit=10  LowerLimit=-10
  Scope : Scope  NumInputPorts=2
  Simulink-PS Converter : nesl_utility/Simulink-PS Converter  PhysicalDomain=network_engine_domain  SubClassName=ps_input  LeftPortType=input  RightPortType=output  PseudoPeriodic=off  Frequencies=[]  NoiseDistribution=none  NoiseParameters=[]  Unit=1  AffineConversion=off  FilteringAndDerivatives=provide  SimscapeFilterOrder=1  InputFilterTimeConstant=0.001  UdotUserProvided=0
  Sum : Sum  Inputs=|-+
  Sum1 : Sum  Inputs=++|
  Sum2 : Sum  Inputs=|++
  Unit Delay1 : UnitDelay  SampleTime=P.Tsc  HasFrameUpgradeWarning=on
  Unit Delay3 : UnitDelay  SampleTime=Ts  HasFrameUpgradeWarning=on
  Variable Resistor : fl_lib/Electrical/Electrical Elements/Variable Resistor  Rmin=0 Ohm  thermalEnable=false  thermal_mass=1 J/K  i_specify=off  i_priority=None  i=0 A  i_nominal_specify=off  i_nominal_unit=A  i_nominal_value=1  v_specify=off  v_priority=None  v=0 V  v_nominal_specify=off  v_nominal_unit=V  v_nominal_value=1  T_specify=off  T_priority=None  T=300 K  T_nominal_specify=off  T_nominal_unit=K  T_nominal_value=1
  Vdc Filter : eeGeneralControl/Low-Pass Filter (Discrete or Continuous)  K=1  T=1e-2  B=inf  A=-inf  init_option=Inherited from block input  x0=0  Ts=P.Tsc
  Voltage Sensor : fl_lib/Electrical/Electrical Sensors/Voltage Sensor
  Zero-Order Hold5 : RateTransition  OutPortSampleTime=P.Tsc
  DCP : PMIOPort  Side=Left
  DCM : PMIOPort  Port=2  Side=Left
  wires:
  Gain4/1 -> Simulink-PS Converter/1
  Saturation1/1 -> Unit Delay1/1
  Saturation/1 -> Gain4/1
  Product/1 -> Unit Delay3/1
  Gain3/1 -> Product/1
  PS-Simulink Converter1/1 -> Gain3/1
  Unit Delay1/1 -> Sum2/2
  Gain2/1 -> Sum2/1
  Gain1/1 -> Sum1/2, Scope/2
  Sum2/1 -> Scope/1, Sum1/1, Saturation1/1
  Sum/1 -> Gain1/1, Gain2/1
  Sum1/1 -> Saturation/1
  Constant/1 -> Sum/2
  Gain/1 -> Product/2
  Vdc Filter/1 -> Sum/1
  Unit Delay3/1 -> Zero-Order Hold5/1
  PS-Simulink Converter3/1 -> Gain/1
  Zero-Order Hold5/1 -> Vdc Filter/1
  connections:
  PS-Simulink Converter1/LConn1 -- Current Sensor/RConn1
  Current Sensor/LConn1 -- Resistor1/RConn1
  Simulink-PS Converter/RConn1 -- Variable Resistor/LConn1
  PS-Simulink Converter3/LConn1 -- Voltage Sensor/RConn1
  Current Sensor/RConn2 -- Voltage Sensor/RConn2 -- DCM/RConn1 -- Variable Resistor/RConn1
  Variable Resistor/LConn2 -- DCP/RConn1 -- Resistor1/LConn1 -- Voltage Sensor/LConn1

== system system_MW/Load_12/Vdc ==
  Voltage Source : ee_lib/Sources/Voltage Source  dc_voltage=P.Udc V  ac_voltage=0 V  ac_shift=0 rad  ac_frequency=fn Hz  noise_mode=ee.enum.sources.noise.Disabled  PSD=0 V^2/Hz  sample_time=1e-3 s  repeatability=ee.enum.sources.repeatability.NotRepeatable  user_seed=0  auto_seed=557942917  i_specify=off  i_priority=None  i=0 A  i_nominal_specify=off  i_nominal_unit=A  i_nominal_value=1  v_specify=off  v_priority=None  v=0 V  v_nominal_specify=off  v_nominal_unit=V  v_nominal_value=1
  DCP : PMIOPort  Side=Left
  DCM : PMIOPort  Port=2  Side=Left
  connections:
  DCM/RConn1 -- Voltage Source/RConn1
  DCP/RConn1 -- Voltage Source/LConn1

== system system_MW/Load_13/Rload ==
  Resistor1 : fl_lib/Electrical/Electrical Elements/Resistor  R=P.Un/P.In/P.p Ohm  i_specify=off  i_priority=None  i=0 A  i_nominal_specify=off  i_nominal_unit=A  i_nominal_value=1  v_specify=off  v_priority=None  v=0 V  v_nominal_specify=off  v_nominal_unit=V  v_nominal_value=1
  DCP : PMIOPort  Side=Left
  DCM : PMIOPort  Port=2  Side=Left
  connections:
  DCP/RConn1 -- Resistor1/LConn1
  DCM/RConn1 -- Resistor1/RConn1

== system system_MW/Load_13/Vdc ==
  Voltage Source : ee_lib/Sources/Voltage Source  dc_voltage=P.Udc V  ac_voltage=0 V  ac_shift=0 rad  ac_frequency=fn Hz  noise_mode=ee.enum.sources.noise.Disabled  PSD=0 V^2/Hz  sample_time=1e-3 s  repeatability=ee.enum.sources.repeatability.NotRepeatable  user_seed=0  auto_seed=2016017452  i_specify=off  i_priority=None  i=0 A  i_nominal_specify=off  i_nominal_unit=A  i_nominal_value=1  v_specify=off  v_priority=None  v=0 V  v_nominal_specify=off  v_nominal_unit=V  v_nominal_value=1
  DCP : PMIOPort  Side=Left
  DCM : PMIOPort  Port=2  Side=Left
  connections:
  DCP/RConn1 -- Voltage Source/LConn1
  DCM/RConn1 -- Voltage Source/RConn1

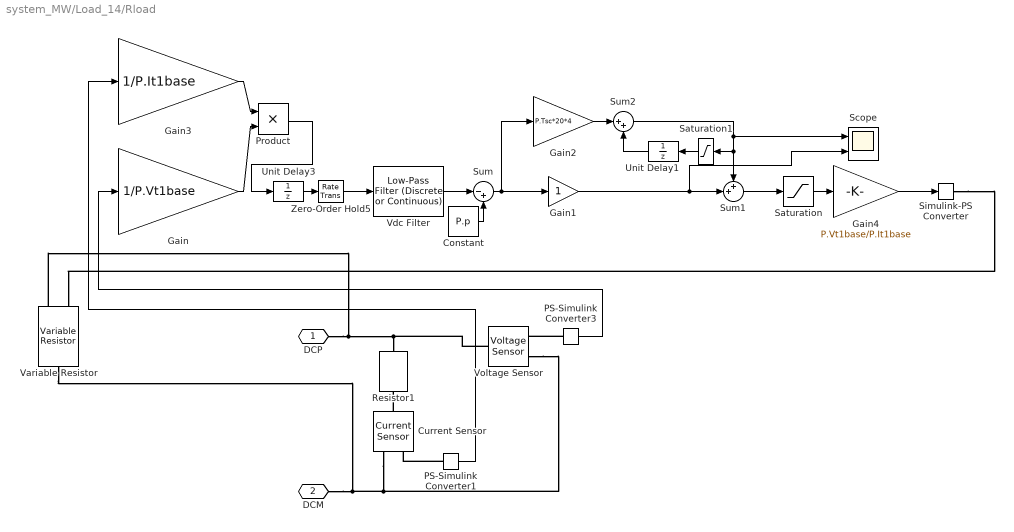
== system system_MW/Load_14/Rload ==
  Constant : Constant  Value=P.p
  Current Sensor : fl_lib/Electrical/Electrical Sensors/Current Sensor
  Gain : Gain  Gain=1/P.Vt1base
  Gain1 : Gain
  Gain2 : Gain  Gain=P.Tsc*20*4
  Gain3 : Gain  Gain=1/P.It1base
  Gain4 : Gain  Gain=P.Vt1base/P.It1base
  PS-Simulink Converter1 : nesl_utility/PS-Simulink Converter  PhysicalDomain=network_engine_domain  SubClassName=ps_output  LeftPortType=input  RightPortType=output  PseudoPeriodic=off  Frequencies=[]  VectorFormat=1-D array  Unit=1  AffineConversion=off
  PS-Simulink Converter3 : nesl_utility/PS-Simulink Converter  PhysicalDomain=network_engine_domain  SubClassName=ps_output  LeftPortType=input  RightPortType=output  PseudoPeriodic=off  Frequencies=[]  VectorFormat=1-D array  Unit=1  AffineConversion=off
  Product : Product
  Resistor1 : fl_lib/Electrical/Electrical Elements/Resistor  R=P.Un/P.In/P.p Ohm  i_specify=off  i_priority=None  i=0 A  i_nominal_specify=off  i_nominal_unit=A  i_nominal_value=1  v_specify=off  v_priority=None  v=0 V  v_nominal_specify=off  v_nominal_unit=V  v_nominal_value=1
  Saturation : Saturate  UpperLimit=10  LowerLimit=-10
  Saturation1 : Saturate  UpperLimit=10  LowerLimit=-10
  Scope : Scope  NumInputPorts=2
  Simulink-PS Converter : nesl_utility/Simulink-PS Converter  PhysicalDomain=network_engine_domain  SubClassName=ps_input  LeftPortType=input  RightPortType=output  PseudoPeriodic=off  Frequencies=[]  NoiseDistribution=none  NoiseParameters=[]  Unit=1  AffineConversion=off  FilteringAndDerivatives=provide  SimscapeFilterOrder=1  InputFilterTimeConstant=0.001  UdotUserProvided=0
  Sum : Sum  Inputs=|-+
  Sum1 : Sum  Inputs=++|
  Sum2 : Sum  Inputs=|++
  Unit Delay1 : UnitDelay  SampleTime=P.Tsc  HasFrameUpgradeWarning=on
  Unit Delay3 : UnitDelay  SampleTime=Ts  HasFrameUpgradeWarning=on
  Variable Resistor : fl_lib/Electrical/Electrical Elements/Variable Resistor  Rmin=0 Ohm  thermalEnable=false  thermal_mass=1 J/K  i_specify=off  i_priority=None  i=0 A  i_nominal_specify=off  i_nominal_unit=A  i_nominal_value=1  v_specify=off  v_priority=None  v=0 V  v_nominal_specify=off  v_nominal_unit=V  v_nominal_value=1  T_specify=off  T_priority=None  T=300 K  T_nominal_specify=off  T_nominal_unit=K  T_nominal_value=1
  Vdc Filter : eeGeneralControl/Low-Pass Filter (Discrete or Continuous)  K=1  T=1e-2  B=inf  A=-inf  init_option=Inherited from block input  x0=0  Ts=P.Tsc
  Voltage Sensor : fl_lib/Electrical/Electrical Sensors/Voltage Sensor
  Zero-Order Hold5 : RateTransition  OutPortSampleTime=P.Tsc
  DCP : PMIOPort  Side=Left
  DCM : PMIOPort  Port=2  Side=Left
  wires:
  Gain4/1 -> Simulink-PS Converter/1
  Saturation1/1 -> Unit Delay1/1
  Saturation/1 -> Gain4/1
  Product/1 -> Unit Delay3/1
  Gain3/1 -> Product/1
  PS-Simulink Converter1/1 -> Gain3/1
  Unit Delay1/1 -> Sum2/2
  Gain2/1 -> Sum2/1
  Gain1/1 -> Sum1/2, Scope/2
  Sum2/1 -> Scope/1, Sum1/1, Saturation1/1
  Sum/1 -> Gain1/1, Gain2/1
  Sum1/1 -> Saturation/1
  Constant/1 -> Sum/2
  Gain/1 -> Product/2
  Vdc Filter/1 -> Sum/1
  Unit Delay3/1 -> Zero-Order Hold5/1
  PS-Simulink Converter3/1 -> Gain/1
  Zero-Order Hold5/1 -> Vdc Filter/1
  connections:
  PS-Simulink Converter1/LConn1 -- Current Sensor/RConn1
  Current Sensor/LConn1 -- Resistor1/RConn1
  Simulink-PS Converter/RConn1 -- Variable Resistor/LConn1
  PS-Simulink Converter3/LConn1 -- Voltage Sensor/RConn1
  Current Sensor/RConn2 -- Voltage Sensor/RConn2 -- DCM/RConn1 -- Variable Resistor/RConn1
  Variable Resistor/LConn2 -- DCP/RConn1 -- Resistor1/LConn1 -- Voltage Sensor/LConn1

== system system_MW/Load_14/Vdc ==
  Voltage Source : ee_lib/Sources/Voltage Source  dc_voltage=P.Udc V  ac_voltage=0 V  ac_shift=0 rad  ac_frequency=fn Hz  noise_mode=ee.enum.sources.noise.Disabled  PSD=0 V^2/Hz  sample_time=1e-3 s  repeatability=ee.enum.sources.repeatability.NotRepeatable  user_seed=0  auto_seed=51119000  i_specify=off  i_priority=None  i=0 A  i_nominal_specify=off  i_nominal_unit=A  i_nominal_value=1  v_specify=off  v_priority=None  v=0 V  v_nominal_specify=off  v_nominal_unit=V  v_nominal_value=1
  DCP : PMIOPort  Side=Left
  DCM : PMIOPort  Port=2  Side=Left
  connections:
  DCM/RConn1 -- Voltage Source/RConn1
  DCP/RConn1 -- Voltage Source/LConn1

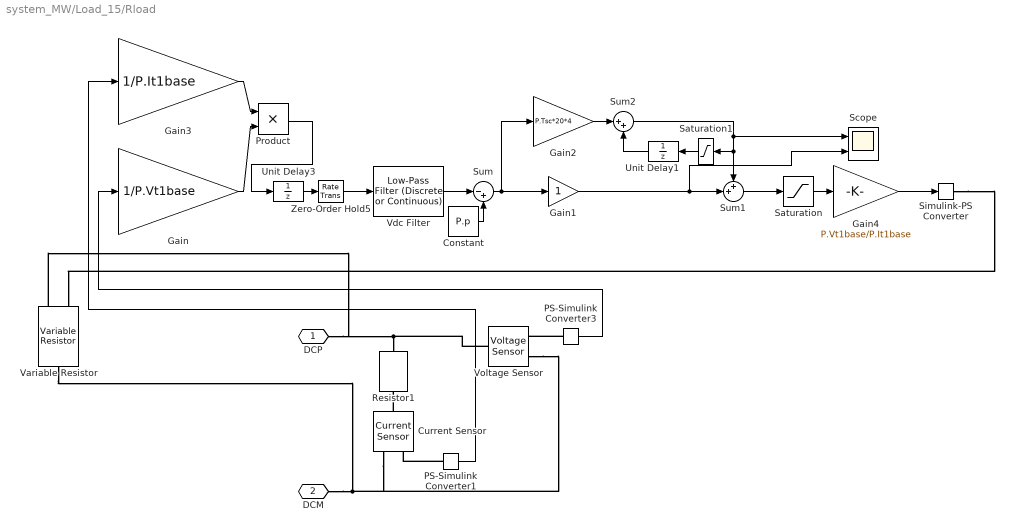
== system system_MW/Load_15/Rload ==
  Constant : Constant  Value=P.p
  Current Sensor : fl_lib/Electrical/Electrical Sensors/Current Sensor
  Gain : Gain  Gain=1/P.Vt1base
  Gain1 : Gain
  Gain2 : Gain  Gain=P.Tsc*20*4
  Gain3 : Gain  Gain=1/P.It1base
  Gain4 : Gain  Gain=P.Vt1base/P.It1base
  PS-Simulink Converter1 : nesl_utility/PS-Simulink Converter  PhysicalDomain=network_engine_domain  SubClassName=ps_output  LeftPortType=input  RightPortType=output  PseudoPeriodic=off  Frequencies=[]  VectorFormat=1-D array  Unit=1  AffineConversion=off
  PS-Simulink Converter3 : nesl_utility/PS-Simulink Converter  PhysicalDomain=network_engine_domain  SubClassName=ps_output  LeftPortType=input  RightPortType=output  PseudoPeriodic=off  Frequencies=[]  VectorFormat=1-D array  Unit=1  AffineConversion=off
  Product : Product
  Resistor1 : fl_lib/Electrical/Electrical Elements/Resistor  R=P.Un/P.In/P.p Ohm  i_specify=off  i_priority=None  i=0 A  i_nominal_specify=off  i_nominal_unit=A  i_nominal_value=1  v_specify=off  v_priority=None  v=0 V  v_nominal_specify=off  v_nominal_unit=V  v_nominal_value=1
  Saturation : Saturate  UpperLimit=10  LowerLimit=-10
  Saturation1 : Saturate  UpperLimit=10  LowerLimit=-10
  Scope : Scope  NumInputPorts=2
  Simulink-PS Converter : nesl_utility/Simulink-PS Converter  PhysicalDomain=network_engine_domain  SubClassName=ps_input  LeftPortType=input  RightPortType=output  PseudoPeriodic=off  Frequencies=[]  NoiseDistribution=none  NoiseParameters=[]  Unit=1  AffineConversion=off  FilteringAndDerivatives=provide  SimscapeFilterOrder=1  InputFilterTimeConstant=0.001  UdotUserProvided=0
  Sum : Sum  Inputs=|-+
  Sum1 : Sum  Inputs=++|
  Sum2 : Sum  Inputs=|++
  Unit Delay1 : UnitDelay  SampleTime=P.Tsc  HasFrameUpgradeWarning=on
  Unit Delay3 : UnitDelay  SampleTime=Ts  HasFrameUpgradeWarning=on
  Variable Resistor : fl_lib/Electrical/Electrical Elements/Variable Resistor  Rmin=0 Ohm  thermalEnable=false  thermal_mass=1 J/K  i_specify=off  i_priority=None  i=0 A  i_nominal_specify=off  i_nominal_unit=A  i_nominal_value=1  v_specify=off  v_priority=None  v=0 V  v_nominal_specify=off  v_nominal_unit=V  v_nominal_value=1  T_specify=off  T_priority=None  T=300 K  T_nominal_specify=off  T_nominal_unit=K  T_nominal_value=1
  Vdc Filter : eeGeneralControl/Low-Pass Filter (Discrete or Continuous)  K=1  T=1e-2  B=inf  A=-inf  init_option=Inherited from block input  x0=0  Ts=P.Tsc
  Voltage Sensor : fl_lib/Electrical/Electrical Sensors/Voltage Sensor
  Zero-Order Hold5 : RateTransition  OutPortSampleTime=P.Tsc
  DCP : PMIOPort  Side=Left
  DCM : PMIOPort  Port=2  Side=Left
  wires:
  Zero-Order Hold5/1 -> Vdc Filter/1
  PS-Simulink Converter3/1 -> Gain/1
  Unit Delay3/1 -> Zero-Order Hold5/1
  Vdc Filter/1 -> Sum/1
  Gain/1 -> Product/2
  Constant/1 -> Sum/2
  Sum1/1 -> Saturation/1
  Sum/1 -> Gain2/1, Gain1/1
  Sum2/1 -> Saturation1/1, Sum1/1, Scope/1
  Gain1/1 -> Scope/2, Sum1/2
  Gain2/1 -> Sum2/1
  Unit Delay1/1 -> Sum2/2
  PS-Simulink Converter1/1 -> Gain3/1
  Gain3/1 -> Product/1
  Product/1 -> Unit Delay3/1
  Saturation/1 -> Gain4/1
  Saturation1/1 -> Unit Delay1/1
  Gain4/1 -> Simulink-PS Converter/1
  connections:
  Voltage Sensor/LConn1 -- Resistor1/LConn1 -- DCP/RConn1 -- Variable Resistor/LConn2
  Variable Resistor/RConn1 -- DCM/RConn1 -- Voltage Sensor/RConn2 -- Current Sensor/RConn2
  PS-Simulink Converter3/LConn1 -- Voltage Sensor/RConn1
  Simulink-PS Converter/RConn1 -- Variable Resistor/LConn1
  Current Sensor/LConn1 -- Resistor1/RConn1
  PS-Simulink Converter1/LConn1 -- Current Sensor/RConn1

== system system_MW/Load_15/Vdc ==
  Voltage Source : ee_lib/Sources/Voltage Source  dc_voltage=P.Udc V  ac_voltage=0 V  ac_shift=0 rad  ac_frequency=fn Hz  noise_mode=ee.enum.sources.noise.Disabled  PSD=0 V^2/Hz  sample_time=1e-3 s  repeatability=ee.enum.sources.repeatability.NotRepeatable  user_seed=0  auto_seed=1447930733  i_specify=off  i_priority=None  i=0 A  i_nominal_specify=off  i_nominal_unit=A  i_nominal_value=1  v_specify=off  v_priority=None  v=0 V  v_nominal_specify=off  v_nominal_unit=V  v_nominal_value=1
  DCP : PMIOPort  Side=Left
  DCM : PMIOPort  Port=2  Side=Left
  connections:
  DCP/RConn1 -- Voltage Source/LConn1
  DCM/RConn1 -- Voltage Source/RConn1

== system system_MW/Load_16/Rload ==
  Resistor1 : fl_lib/Electrical/Electrical Elements/Resistor  R=P.Un/P.In/P.p Ohm  i_specify=off  i_priority=None  i=0 A  i_nominal_specify=off  i_nominal_unit=A  i_nominal_value=1  v_specify=off  v_priority=None  v=0 V  v_nominal_specify=off  v_nominal_unit=V  v_nominal_value=1
  DCP : PMIOPort  Side=Left
  DCM : PMIOPort  Port=2  Side=Left
  connections:
  DCM/RConn1 -- Resistor1/RConn1
  DCP/RConn1 -- Resistor1/LConn1

== system system_MW/Load_16/Vdc ==
  Voltage Source : ee_lib/Sources/Voltage Source  dc_voltage=P.Udc V  ac_voltage=0 V  ac_shift=0 rad  ac_frequency=fn Hz  noise_mode=ee.enum.sources.noise.Disabled  PSD=0 V^2/Hz  sample_time=1e-3 s  repeatability=ee.enum.sources.repeatability.NotRepeatable  user_seed=0  auto_seed=696567710  i_specify=off  i_priority=None  i=0 A  i_nominal_specify=off  i_nominal_unit=A  i_nominal_value=1  v_specify=off  v_priority=None  v=0 V  v_nominal_specify=off  v_nominal_unit=V  v_nominal_value=1
  DCP : PMIOPort  Side=Left
  DCM : PMIOPort  Port=2  Side=Left
  connections:
  DCM/RConn1 -- Voltage Source/RConn1
  DCP/RConn1 -- Voltage Source/LConn1

== system system_MW/Load_17/Rload ==
  Resistor1 : fl_lib/Electrical/Electrical Elements/Resistor  R=P.Un/P.In/P.p Ohm  i_specify=off  i_priority=None  i=0 A  i_nominal_specify=off  i_nominal_unit=A  i_nominal_value=1  v_specify=off  v_priority=None  v=0 V  v_nominal_specify=off  v_nominal_unit=V  v_nominal_value=1
  DCP : PMIOPort  Side=Left
  DCM : PMIOPort  Port=2  Side=Left
  connections:
  DCM/RConn1 -- Resistor1/RConn1
  DCP/RConn1 -- Resistor1/LConn1

== system system_MW/Load_17/Vdc ==
  Voltage Source : ee_lib/Sources/Voltage Source  dc_voltage=P.Udc V  ac_voltage=0 V  ac_shift=0 rad  ac_frequency=fn Hz  noise_mode=ee.enum.sources.noise.Disabled  PSD=0 V^2/Hz  sample_time=1e-3 s  repeatability=ee.enum.sources.repeatability.NotRepeatable  user_seed=0  auto_seed=3411426126  i_specify=off  i_priority=None  i=0 A  i_nominal_specify=off  i_nominal_unit=A  i_nominal_value=1  v_specify=off  v_priority=None  v=0 V  v_nominal_specify=off  v_nominal_unit=V  v_nominal_value=1
  DCP : PMIOPort  Side=Left
  DCM : PMIOPort  Port=2  Side=Left
  connections:
  DCM/RConn1 -- Voltage Source/RConn1
  DCP/RConn1 -- Voltage Source/LConn1
